simulink model "generalModelForErrorsNEW"  (R2016b)
settings: Solver=ode15s  StartTime=0  StopTime=3500  FixedStep=0.0001  MaxStep=0.001  RelTol=1e-3
values from neighbouring files (symbols this model uses):
  bigpump_const = 1    [run_model.m]
  gain_coef = 4000*10    (= 40000)    [params.m]    (also in run_model.m)
  min_vol = 20    [params.m]
  minipump_const = 0    [run_model.m]
  pipe_diameter = 2    [params.m]
  pressurization = 100000    [params.m]
  pump_speed = 20000    [params.m]
  valve_gain = 0.01    [params.m]
  ws_fault_time = fault_time    [run_model.m]
  ws_sample_time_end_valve_bigpump_in = 0    [run_model.m]
  ws_sample_time_end_valve_bigpump_out = 0    [run_model.m]
  ws_sample_time_end_valve_car_tank = 0    [run_model.m]
  ws_sample_time_end_valve_cartank1_in = 0    [run_model.m]
  ws_sample_time_end_valve_cartank1_out = 0    [run_model.m]
  ws_sample_time_end_valve_cartank2_in = 0    [run_model.m]
  ws_sample_time_end_valve_cartank2_out = 0    [run_model.m]
  ws_sample_time_end_valve_cartank3_in = 0    [run_model.m]
  ws_sample_time_end_valve_cartank3_out = 0    [run_model.m]
  ws_sample_time_end_valve_general_tank = 0    [run_model.m]
  ws_sample_time_end_valve_minipump_in = 0    [run_model.m]
  ws_sample_time_end_valve_minipump_out = 0    [run_model.m]
undefined symbols (not defined in the file or in its folder): sigbuilder_block
libraries: sh_lib x61, nesl_utility x34, fl_lib x32, powerlib_meascontrol x2
(part 2 of 2)

== system generalModelForErrorsNEW/Bigpump/Valve Control3 ==
  In1 : Inport
  Constant : Constant  Value=ws_sample_time_end_valve_bigpump_out
  Logical Operator : Logic  AllPortsSameDT=off  OutDataTypeStr=boolean
  Product : Product
  S2PS1 : nesl_utility/Simulink-PS Converter  PhysicalDomain=network_engine_domain  SubClassName=ps_input  LeftPortType=input  RightPortType=output  PseudoPeriodic=off  Frequencies=[]  NoiseDistribution=none  NoiseParameters=[]  Unit=1  AffineConversion=off  InputFiltering=off  SimscapeFilterOrder=1  InputFilterTimeConstant=.001  UdotUserProvided=0
  Signal Builder : Subsystem  Tag=STV Subsys  LoadFcn=sigbuilder_block('load');  StartFcn=sigbuilder_block('start');  StopFcn=sigbuilder_block('stop');  ClipboardFcn=sigbuilder_block('clipboard');  mask(Sigbuilder block){tuvar=[0:10]}
      mask help: Simulink:masks:SigbuilderBlock_MD
      mask init:
      | if ~strcmp(get_param(bdroot(gcbh),'SimulationStatus'),'stopped') tuvar = sigbuilder_block('maskInit'); end
      settings: CopyFcn=sigbuilder_block('copy');  DeleteFcn=sigbuilder_block('delete');  ModelCloseFcn=sigbuilder_block('modelClose');  PreSaveFcn=sigbuilder_block('preSave');  PauseFcn=sigbuilder_block('pause');  ContinueFcn=sigbuilder_block('continue');  NameChangeFcn=sigbuilder_block('namechange');  OpenFcn=sigbuilder_block('open',[1024.5 -234 1440 722.25 ]);  CloseFcn=sigbuilder_block('close');
      mask Display: plot(0, 0, 100, 100,[2, 2, 32, 32, 2], [68, 8, 8, 68, 68],[32, 2], [38, 38], [32, 19, 2],[53, 60, 44], [32, 17, 17, 2],[16, 16, 31, 31]);txt = getActiveGroup(gcbh);text(2, 100, txt,'verticalAlignment', 'top');
  Transport Delay : TransportDelay  DelayTime=ws_fault_time
  Valve Actuator : sh_lib/Valves/Valve Actuators/Valve Actuator  valve_stroke=valve_stroke m  time_constant=0.01 s  gain=valve_gain*5 m
  Signal : PMIOPort  Port=1  Side=Left
  wires:
  Product/1 -> S2PS1/1
  In1/1 -> Logical Operator/1
  Signal Builder/1(Signal 2) -> Transport Delay/1
  Transport Delay/1 -> Product/2
  Constant/1 -> Logical Operator/2
  Logical Operator/1 -> Product/1
  connections:
  Valve Actuator/RConn1 -- Signal/RConn1
  Valve Actuator/LConn1 -- S2PS1/RConn1

== system generalModelForErrorsNEW/Bigpump/pressure sensor ==
  Hydraulic Pressure Sensor1 : fl_lib/Hydraulic/Hydraulic Sensors/Hydraulic Pressure Sensor
  Hydraulic Reference : fl_lib/Hydraulic/Hydraulic Elements/Hydraulic Reference
  PS-Simulink Converter1 : nesl_utility/PS-Simulink Converter  PhysicalDomain=network_engine_domain  SubClassName=ps_output  LeftPortType=input  RightPortType=output  PseudoPeriodic=off  Frequencies=[]  Unit=1  AffineConversion=off
  Connection Port : PMIOPort  Port=1  Side=Left
  Pressure_valve_bigpump_out : Outport
  wires:
  PS-Simulink Converter1/1 -> Pressure_valve_bigpump_out/1
  connections:
  PS-Simulink Converter1/LConn1 -- Hydraulic Pressure Sensor1/RConn2
  Hydraulic Reference/LConn1 -- Hydraulic Pressure Sensor1/RConn1
  Connection Port/RConn1 -- Hydraulic Pressure Sensor1/LConn1

== system generalModelForErrorsNEW/Bigpump/pressure sensor1 ==
  Hydraulic Pressure Sensor1 : fl_lib/Hydraulic/Hydraulic Sensors/Hydraulic Pressure Sensor
  Hydraulic Reference : fl_lib/Hydraulic/Hydraulic Elements/Hydraulic Reference
  PS-Simulink Converter1 : nesl_utility/PS-Simulink Converter  PhysicalDomain=network_engine_domain  SubClassName=ps_output  LeftPortType=input  RightPortType=output  PseudoPeriodic=off  Frequencies=[]  Unit=1  AffineConversion=off
  Connection Port : PMIOPort  Port=1  Side=Left
  Pressure_valve_bigpump_in : Outport
  wires:
  PS-Simulink Converter1/1 -> Pressure_valve_bigpump_in/1
  connections:
  PS-Simulink Converter1/LConn1 -- Hydraulic Pressure Sensor1/RConn2
  Hydraulic Reference/LConn1 -- Hydraulic Pressure Sensor1/RConn1
  Connection Port/RConn1 -- Hydraulic Pressure Sensor1/LConn1

== system generalModelForErrorsNEW/Car_Tank/Valve Control ==
  In1 : Inport
  Constant : Constant  Value=ws_sample_time_end_valve_car_tank
  Logical Operator : Logic  AllPortsSameDT=off  OutDataTypeStr=boolean
  Product : Product
  S2PS1 : nesl_utility/Simulink-PS Converter  PhysicalDomain=network_engine_domain  SubClassName=ps_input  LeftPortType=input  RightPortType=output  PseudoPeriodic=off  Frequencies=[]  NoiseDistribution=none  NoiseParameters=[]  Unit=1  AffineConversion=off  InputFiltering=off  SimscapeFilterOrder=1  InputFilterTimeConstant=.001  UdotUserProvided=0
  Scope : Scope
  Scope1 : Scope
  Signal Builder : Subsystem  Tag=STV Subsys  LoadFcn=sigbuilder_block('load');  StartFcn=sigbuilder_block('start');  StopFcn=sigbuilder_block('stop');  ClipboardFcn=sigbuilder_block('clipboard');  mask(Sigbuilder block){tuvar=[0:10]}
      mask help: Simulink:masks:SigbuilderBlock_MD
      mask init:
      | if ~strcmp(get_param(bdroot(gcbh),'SimulationStatus'),'stopped') tuvar = sigbuilder_block('maskInit'); end
      settings: CopyFcn=sigbuilder_block('copy');  DeleteFcn=sigbuilder_block('delete');  ModelCloseFcn=sigbuilder_block('modelClose');  PreSaveFcn=sigbuilder_block('preSave');  PauseFcn=sigbuilder_block('pause');  ContinueFcn=sigbuilder_block('continue');  NameChangeFcn=sigbuilder_block('namechange');  OpenFcn=sigbuilder_block('open',[1024.5 -234 1440 722.25 ]);  CloseFcn=sigbuilder_block('close');
      mask Display: plot(0, 0, 100, 100,[2, 2, 32, 32, 2], [68, 8, 8, 68, 68],[32, 2], [38, 38], [32, 19, 2],[53, 60, 44], [32, 17, 17, 2],[16, 16, 31, 31]);txt = getActiveGroup(gcbh);text(2, 100, txt,'verticalAlignment', 'top');
  Transport Delay : TransportDelay  DelayTime=ws_fault_time
  Valve Actuator : sh_lib/Valves/Valve Actuators/Valve Actuator  valve_stroke=valve_stroke m  time_constant=0.01 s  gain=valve_gain*5 m
  Signal : PMIOPort  Port=1  Side=Left
  wires:
  Product/1 -> Scope1/1, S2PS1/1
  Signal Builder/1(Signal 2) -> Transport Delay/1
  Transport Delay/1 -> Product/2
  In1/1 -> Logical Operator/1
  Constant/1 -> Logical Operator/2
  Logical Operator/1 -> Scope/1, Product/1
  connections:
  Valve Actuator/RConn1 -- Signal/RConn1
  Valve Actuator/LConn1 -- S2PS1/RConn1

== system generalModelForErrorsNEW/General_TANK/Valve Control2 ==
  In1 : Inport
  Constant : Constant  Value=ws_sample_time_end_valve_general_tank
  Logical Operator : Logic  AllPortsSameDT=off  OutDataTypeStr=boolean
  Product : Product
  S2PS1 : nesl_utility/Simulink-PS Converter  PhysicalDomain=network_engine_domain  SubClassName=ps_input  LeftPortType=input  RightPortType=output  PseudoPeriodic=off  Frequencies=[]  NoiseDistribution=none  NoiseParameters=[]  Unit=1  AffineConversion=off  InputFiltering=off  SimscapeFilterOrder=1  InputFilterTimeConstant=.001  UdotUserProvided=0
  Signal Builder : Subsystem  Tag=STV Subsys  LoadFcn=sigbuilder_block('load');  StartFcn=sigbuilder_block('start');  StopFcn=sigbuilder_block('stop');  ClipboardFcn=sigbuilder_block('clipboard');  mask(Sigbuilder block){tuvar=[0:10]}
      mask help: Simulink:masks:SigbuilderBlock_MD
      mask init:
      | if ~strcmp(get_param(bdroot(gcbh),'SimulationStatus'),'stopped') tuvar = sigbuilder_block('maskInit'); end
      settings: CopyFcn=sigbuilder_block('copy');  DeleteFcn=sigbuilder_block('delete');  ModelCloseFcn=sigbuilder_block('modelClose');  PreSaveFcn=sigbuilder_block('preSave');  PauseFcn=sigbuilder_block('pause');  ContinueFcn=sigbuilder_block('continue');  NameChangeFcn=sigbuilder_block('namechange');  OpenFcn=sigbuilder_block('open',[1024.5 -234 1440 722.25 ]);  CloseFcn=sigbuilder_block('close');
      mask Display: plot(0, 0, 100, 100,[2, 2, 32, 32, 2], [68, 8, 8, 68, 68],[32, 2], [38, 38], [32, 19, 2],[53, 60, 44], [32, 17, 17, 2],[16, 16, 31, 31]);txt = getActiveGroup(gcbh);text(2, 100, txt,'verticalAlignment', 'top');
  Transport Delay : TransportDelay  DelayTime=ws_fault_time
  Valve Actuator : sh_lib/Valves/Valve Actuators/Valve Actuator  valve_stroke=valve_stroke m  time_constant=0.01 s  gain=valve_gain*5 m
  Signal : PMIOPort  Port=1  Side=Left
  wires:
  Product/1 -> S2PS1/1
  In1/1 -> Logical Operator/1
  Signal Builder/1(Signal 2) -> Transport Delay/1
  Transport Delay/1 -> Product/2
  Constant/1 -> Logical Operator/2
  Logical Operator/1 -> Product/1
  connections:
  Valve Actuator/RConn1 -- Signal/RConn1
  Valve Actuator/LConn1 -- S2PS1/RConn1

== system generalModelForErrorsNEW/Tank1/Valve Control1 ==
  In1 : Inport
  Constant : Constant  Value=ws_sample_time_end_valve_cartank1_in
  Logical Operator : Logic  AllPortsSameDT=off  OutDataTypeStr=boolean
  Product : Product
  S2PS1 : nesl_utility/Simulink-PS Converter  PhysicalDomain=network_engine_domain  SubClassName=ps_input  LeftPortType=input  RightPortType=output  PseudoPeriodic=off  Frequencies=[]  NoiseDistribution=none  NoiseParameters=[]  Unit=1  AffineConversion=off  InputFiltering=off  SimscapeFilterOrder=1  InputFilterTimeConstant=.001  UdotUserProvided=0
  Signal Builder : Subsystem  Tag=STV Subsys  LoadFcn=sigbuilder_block('load');  StartFcn=sigbuilder_block('start');  StopFcn=sigbuilder_block('stop');  ClipboardFcn=sigbuilder_block('clipboard');  mask(Sigbuilder block){tuvar=[0:10]}
      mask help: Simulink:masks:SigbuilderBlock_MD
      mask init:
      | if ~strcmp(get_param(bdroot(gcbh),'SimulationStatus'),'stopped') tuvar = sigbuilder_block('maskInit'); end
      settings: CopyFcn=sigbuilder_block('copy');  DeleteFcn=sigbuilder_block('delete');  ModelCloseFcn=sigbuilder_block('modelClose');  PreSaveFcn=sigbuilder_block('preSave');  PauseFcn=sigbuilder_block('pause');  ContinueFcn=sigbuilder_block('continue');  NameChangeFcn=sigbuilder_block('namechange');  OpenFcn=sigbuilder_block('open',[1024.5 -234 1440 722.25 ]);  CloseFcn=sigbuilder_block('close');
      mask Display: plot(0, 0, 100, 100,[2, 2, 32, 32, 2], [68, 8, 8, 68, 68],[32, 2], [38, 38], [32, 19, 2],[53, 60, 44], [32, 17, 17, 2],[16, 16, 31, 31]);txt = getActiveGroup(gcbh);text(2, 100, txt,'verticalAlignment', 'top');
  Transport Delay : TransportDelay  DelayTime=ws_fault_time
  Valve Actuator : sh_lib/Valves/Valve Actuators/Valve Actuator  valve_stroke=valve_stroke m  time_constant=0.01 s  gain=valve_gain*5 m
  Signal : PMIOPort  Port=1  Side=Left
  wires:
  Product/1 -> S2PS1/1
  In1/1 -> Logical Operator/1
  Signal Builder/1(Signal 2) -> Transport Delay/1
  Transport Delay/1 -> Product/2
  Constant/1 -> Logical Operator/2
  Logical Operator/1 -> Product/1
  connections:
  Valve Actuator/RConn1 -- Signal/RConn1
  Valve Actuator/LConn1 -- S2PS1/RConn1

== system generalModelForErrorsNEW/Tank1/Valve Control2 ==
  In1 : Inport
  Constant : Constant  Value=ws_sample_time_end_valve_cartank1_out
  Logical Operator : Logic  AllPortsSameDT=off  OutDataTypeStr=boolean
  Product : Product
  S2PS1 : nesl_utility/Simulink-PS Converter  PhysicalDomain=network_engine_domain  SubClassName=ps_input  LeftPortType=input  RightPortType=output  PseudoPeriodic=off  Frequencies=[]  NoiseDistribution=none  NoiseParameters=[]  Unit=1  AffineConversion=off  InputFiltering=off  SimscapeFilterOrder=1  InputFilterTimeConstant=.001  UdotUserProvided=0
  Signal Builder : Subsystem  Tag=STV Subsys  LoadFcn=sigbuilder_block('load');  StartFcn=sigbuilder_block('start');  StopFcn=sigbuilder_block('stop');  ClipboardFcn=sigbuilder_block('clipboard');  mask(Sigbuilder block){tuvar=[0:10]}
      mask help: Simulink:masks:SigbuilderBlock_MD
      mask init:
      | if ~strcmp(get_param(bdroot(gcbh),'SimulationStatus'),'stopped') tuvar = sigbuilder_block('maskInit'); end
      settings: CopyFcn=sigbuilder_block('copy');  DeleteFcn=sigbuilder_block('delete');  ModelCloseFcn=sigbuilder_block('modelClose');  PreSaveFcn=sigbuilder_block('preSave');  PauseFcn=sigbuilder_block('pause');  ContinueFcn=sigbuilder_block('continue');  NameChangeFcn=sigbuilder_block('namechange');  OpenFcn=sigbuilder_block('open',[1024.5 -234 1440 722.25 ]);  CloseFcn=sigbuilder_block('close');
      mask Display: plot(0, 0, 100, 100,[2, 2, 32, 32, 2], [68, 8, 8, 68, 68],[32, 2], [38, 38], [32, 19, 2],[53, 60, 44], [32, 17, 17, 2],[16, 16, 31, 31]);txt = getActiveGroup(gcbh);text(2, 100, txt,'verticalAlignment', 'top');
  Transport Delay : TransportDelay  DelayTime=ws_fault_time
  Valve Actuator : sh_lib/Valves/Valve Actuators/Valve Actuator  valve_stroke=valve_stroke m  time_constant=0.01 s  gain=valve_gain*5 m
  Signal : PMIOPort  Port=1  Side=Left
  wires:
  Product/1 -> S2PS1/1
  In1/1 -> Logical Operator/1
  Signal Builder/1(Signal 2) -> Transport Delay/1
  Transport Delay/1 -> Product/2
  Constant/1 -> Logical Operator/2
  Logical Operator/1 -> Product/1
  connections:
  Valve Actuator/RConn1 -- Signal/RConn1
  Valve Actuator/LConn1 -- S2PS1/RConn1

== system generalModelForErrorsNEW/Tank2/Valve Control1 ==
  In1 : Inport
  Constant : Constant  Value=ws_sample_time_end_valve_cartank2_in
  Logical Operator : Logic  AllPortsSameDT=off  OutDataTypeStr=boolean
  Product : Product
  S2PS1 : nesl_utility/Simulink-PS Converter  PhysicalDomain=network_engine_domain  SubClassName=ps_input  LeftPortType=input  RightPortType=output  PseudoPeriodic=off  Frequencies=[]  NoiseDistribution=none  NoiseParameters=[]  Unit=1  AffineConversion=off  InputFiltering=off  SimscapeFilterOrder=1  InputFilterTimeConstant=.001  UdotUserProvided=0
  Signal Builder : Subsystem  Tag=STV Subsys  LoadFcn=sigbuilder_block('load');  StartFcn=sigbuilder_block('start');  StopFcn=sigbuilder_block('stop');  ClipboardFcn=sigbuilder_block('clipboard');  mask(Sigbuilder block){tuvar=[0:10]}
      mask help: Simulink:masks:SigbuilderBlock_MD
      mask init:
      | if ~strcmp(get_param(bdroot(gcbh),'SimulationStatus'),'stopped') tuvar = sigbuilder_block('maskInit'); end
      settings: CopyFcn=sigbuilder_block('copy');  DeleteFcn=sigbuilder_block('delete');  ModelCloseFcn=sigbuilder_block('modelClose');  PreSaveFcn=sigbuilder_block('preSave');  PauseFcn=sigbuilder_block('pause');  ContinueFcn=sigbuilder_block('continue');  NameChangeFcn=sigbuilder_block('namechange');  OpenFcn=sigbuilder_block('open',[1024.5 -234 1440 722.25 ]);  CloseFcn=sigbuilder_block('close');
      mask Display: plot(0, 0, 100, 100,[2, 2, 32, 32, 2], [68, 8, 8, 68, 68],[32, 2], [38, 38], [32, 19, 2],[53, 60, 44], [32, 17, 17, 2],[16, 16, 31, 31]);txt = getActiveGroup(gcbh);text(2, 100, txt,'verticalAlignment', 'top');
  Transport Delay : TransportDelay  DelayTime=ws_fault_time
  Valve Actuator : sh_lib/Valves/Valve Actuators/Valve Actuator  valve_stroke=valve_stroke m  time_constant=0.01 s  gain=valve_gain*5 m
  Signal : PMIOPort  Port=1  Side=Left
  wires:
  Product/1 -> S2PS1/1
  In1/1 -> Logical Operator/1
  Signal Builder/1(Signal 2) -> Transport Delay/1
  Transport Delay/1 -> Product/2
  Constant/1 -> Logical Operator/2
  Logical Operator/1 -> Product/1
  connections:
  Valve Actuator/RConn1 -- Signal/RConn1
  Valve Actuator/LConn1 -- S2PS1/RConn1

== system generalModelForErrorsNEW/Tank2/Valve Control2 ==
  In1 : Inport
  Constant : Constant  Value=ws_sample_time_end_valve_cartank2_out
  Logical Operator : Logic  AllPortsSameDT=off  OutDataTypeStr=boolean
  Product : Product
  S2PS1 : nesl_utility/Simulink-PS Converter  PhysicalDomain=network_engine_domain  SubClassName=ps_input  LeftPortType=input  RightPortType=output  PseudoPeriodic=off  Frequencies=[]  NoiseDistribution=none  NoiseParameters=[]  Unit=1  AffineConversion=off  InputFiltering=off  SimscapeFilterOrder=1  InputFilterTimeConstant=.001  UdotUserProvided=0
  Signal Builder : Subsystem  Tag=STV Subsys  LoadFcn=sigbuilder_block('load');  StartFcn=sigbuilder_block('start');  StopFcn=sigbuilder_block('stop');  ClipboardFcn=sigbuilder_block('clipboard');  mask(Sigbuilder block){tuvar=[0:10]}
      mask help: Simulink:masks:SigbuilderBlock_MD
      mask init:
      | if ~strcmp(get_param(bdroot(gcbh),'SimulationStatus'),'stopped') tuvar = sigbuilder_block('maskInit'); end
      settings: CopyFcn=sigbuilder_block('copy');  DeleteFcn=sigbuilder_block('delete');  ModelCloseFcn=sigbuilder_block('modelClose');  PreSaveFcn=sigbuilder_block('preSave');  PauseFcn=sigbuilder_block('pause');  ContinueFcn=sigbuilder_block('continue');  NameChangeFcn=sigbuilder_block('namechange');  OpenFcn=sigbuilder_block('open',[1024.5 -234 1440 722.25 ]);  CloseFcn=sigbuilder_block('close');
      mask Display: plot(0, 0, 100, 100,[2, 2, 32, 32, 2], [68, 8, 8, 68, 68],[32, 2], [38, 38], [32, 19, 2],[53, 60, 44], [32, 17, 17, 2],[16, 16, 31, 31]);txt = getActiveGroup(gcbh);text(2, 100, txt,'verticalAlignment', 'top');
  Transport Delay : TransportDelay  DelayTime=ws_fault_time
  Valve Actuator : sh_lib/Valves/Valve Actuators/Valve Actuator  valve_stroke=valve_stroke m  time_constant=0.01 s  gain=valve_gain*5 m
  Signal : PMIOPort  Port=1  Side=Left
  wires:
  Product/1 -> S2PS1/1
  In1/1 -> Logical Operator/1
  Signal Builder/1(Signal 2) -> Transport Delay/1
  Transport Delay/1 -> Product/2
  Constant/1 -> Logical Operator/2
  Logical Operator/1 -> Product/1
  connections:
  Valve Actuator/RConn1 -- Signal/RConn1
  Valve Actuator/LConn1 -- S2PS1/RConn1

== system generalModelForErrorsNEW/Tank3/Valve Control1 ==
  In1 : Inport
  Constant : Constant  Value=ws_sample_time_end_valve_cartank3_out
  Logical Operator : Logic  AllPortsSameDT=off  OutDataTypeStr=boolean
  Product : Product
  S2PS1 : nesl_utility/Simulink-PS Converter  PhysicalDomain=network_engine_domain  SubClassName=ps_input  LeftPortType=input  RightPortType=output  PseudoPeriodic=off  Frequencies=[]  NoiseDistribution=none  NoiseParameters=[]  Unit=1  AffineConversion=off  InputFiltering=off  SimscapeFilterOrder=1  InputFilterTimeConstant=.001  UdotUserProvided=0
  Signal Builder : Subsystem  Tag=STV Subsys  LoadFcn=sigbuilder_block('load');  StartFcn=sigbuilder_block('start');  StopFcn=sigbuilder_block('stop');  ClipboardFcn=sigbuilder_block('clipboard');  mask(Sigbuilder block){tuvar=[0:10]}
      mask help: Simulink:masks:SigbuilderBlock_MD
      mask init:
      | if ~strcmp(get_param(bdroot(gcbh),'SimulationStatus'),'stopped') tuvar = sigbuilder_block('maskInit'); end
      settings: CopyFcn=sigbuilder_block('copy');  DeleteFcn=sigbuilder_block('delete');  ModelCloseFcn=sigbuilder_block('modelClose');  PreSaveFcn=sigbuilder_block('preSave');  PauseFcn=sigbuilder_block('pause');  ContinueFcn=sigbuilder_block('continue');  NameChangeFcn=sigbuilder_block('namechange');  OpenFcn=sigbuilder_block('open',[1024.5 -234 1440 722.25 ]);  CloseFcn=sigbuilder_block('close');
      mask Display: plot(0, 0, 100, 100,[2, 2, 32, 32, 2], [68, 8, 8, 68, 68],[32, 2], [38, 38], [32, 19, 2],[53, 60, 44], [32, 17, 17, 2],[16, 16, 31, 31]);txt = getActiveGroup(gcbh);text(2, 100, txt,'verticalAlignment', 'top');
  Transport Delay : TransportDelay  DelayTime=ws_fault_time
  Valve Actuator : sh_lib/Valves/Valve Actuators/Valve Actuator  valve_stroke=valve_stroke m  time_constant=0.01 s  gain=valve_gain*5 m
  Signal : PMIOPort  Port=1  Side=Left
  wires:
  Product/1 -> S2PS1/1
  In1/1 -> Logical Operator/1
  Signal Builder/1(Signal 2) -> Transport Delay/1
  Transport Delay/1 -> Product/2
  Constant/1 -> Logical Operator/2
  Logical Operator/1 -> Product/1
  connections:
  Valve Actuator/RConn1 -- Signal/RConn1
  Valve Actuator/LConn1 -- S2PS1/RConn1

== system generalModelForErrorsNEW/Tank3/Valve Control2 ==
  In1 : Inport
  Constant : Constant  Value=ws_sample_time_end_valve_cartank3_in
  Logical Operator : Logic  AllPortsSameDT=off  OutDataTypeStr=boolean
  Product : Product
  S2PS1 : nesl_utility/Simulink-PS Converter  PhysicalDomain=network_engine_domain  SubClassName=ps_input  LeftPortType=input  RightPortType=output  PseudoPeriodic=off  Frequencies=[]  NoiseDistribution=none  NoiseParameters=[]  Unit=1  AffineConversion=off  InputFiltering=off  SimscapeFilterOrder=1  InputFilterTimeConstant=.001  UdotUserProvided=0
  Signal Builder : Subsystem  Tag=STV Subsys  LoadFcn=sigbuilder_block('load');  StartFcn=sigbuilder_block('start');  StopFcn=sigbuilder_block('stop');  ClipboardFcn=sigbuilder_block('clipboard');  mask(Sigbuilder block){tuvar=[0:10]}
      mask help: Simulink:masks:SigbuilderBlock_MD
      mask init:
      | if ~strcmp(get_param(bdroot(gcbh),'SimulationStatus'),'stopped') tuvar = sigbuilder_block('maskInit'); end
      settings: CopyFcn=sigbuilder_block('copy');  DeleteFcn=sigbuilder_block('delete');  ModelCloseFcn=sigbuilder_block('modelClose');  PreSaveFcn=sigbuilder_block('preSave');  PauseFcn=sigbuilder_block('pause');  ContinueFcn=sigbuilder_block('continue');  NameChangeFcn=sigbuilder_block('namechange');  OpenFcn=sigbuilder_block('open',[1024.5 -234 1440 722.25 ]);  CloseFcn=sigbuilder_block('close');
      mask Display: plot(0, 0, 100, 100,[2, 2, 32, 32, 2], [68, 8, 8, 68, 68],[32, 2], [38, 38], [32, 19, 2],[53, 60, 44], [32, 17, 17, 2],[16, 16, 31, 31]);txt = getActiveGroup(gcbh);text(2, 100, txt,'verticalAlignment', 'top');
  Transport Delay : TransportDelay  DelayTime=ws_fault_time
  Valve Actuator : sh_lib/Valves/Valve Actuators/Valve Actuator  valve_stroke=valve_stroke m  time_constant=0.01 s  gain=valve_gain*5 m
  Signal : PMIOPort  Port=1  Side=Left
  wires:
  Product/1 -> S2PS1/1
  In1/1 -> Logical Operator/1
  Signal Builder/1(Signal 2) -> Transport Delay/1
  Transport Delay/1 -> Product/2
  Constant/1 -> Logical Operator/2
  Logical Operator/1 -> Product/1
  connections:
  Valve Actuator/RConn1 -- Signal/RConn1
  Valve Actuator/LConn1 -- S2PS1/RConn1

== system generalModelForErrorsNEW/minipump/Pressure sensor1 ==
  Hydraulic Pressure Sensor1 : fl_lib/Hydraulic/Hydraulic Sensors/Hydraulic Pressure Sensor
  Hydraulic Reference : fl_lib/Hydraulic/Hydraulic Elements/Hydraulic Reference
  PS-Simulink Converter1 : nesl_utility/PS-Simulink Converter  PhysicalDomain=network_engine_domain  SubClassName=ps_output  LeftPortType=input  RightPortType=output  PseudoPeriodic=off  Frequencies=[]  Unit=1  AffineConversion=off
  Connection Port : PMIOPort  Port=1  Side=Left
  Pressure_valve_pump_out : Outport
  wires:
  PS-Simulink Converter1/1 -> Pressure_valve_pump_out/1
  connections:
  PS-Simulink Converter1/LConn1 -- Hydraulic Pressure Sensor1/RConn2
  Hydraulic Reference/LConn1 -- Hydraulic Pressure Sensor1/RConn1
  Connection Port/RConn1 -- Hydraulic Pressure Sensor1/LConn1

== system generalModelForErrorsNEW/minipump/Pressure sensor2 ==
  Hydraulic Pressure Sensor1 : fl_lib/Hydraulic/Hydraulic Sensors/Hydraulic Pressure Sensor
  Hydraulic Reference : fl_lib/Hydraulic/Hydraulic Elements/Hydraulic Reference
  PS-Simulink Converter1 : nesl_utility/PS-Simulink Converter  PhysicalDomain=network_engine_domain  SubClassName=ps_output  LeftPortType=input  RightPortType=output  PseudoPeriodic=off  Frequencies=[]  Unit=1  AffineConversion=off
  Connection Port : PMIOPort  Port=1  Side=Left
  Pressure_valve_pump_in : Outport
  wires:
  PS-Simulink Converter1/1 -> Pressure_valve_pump_in/1
  connections:
  PS-Simulink Converter1/LConn1 -- Hydraulic Pressure Sensor1/RConn2
  Hydraulic Reference/LConn1 -- Hydraulic Pressure Sensor1/RConn1
  Connection Port/RConn1 -- Hydraulic Pressure Sensor1/LConn1

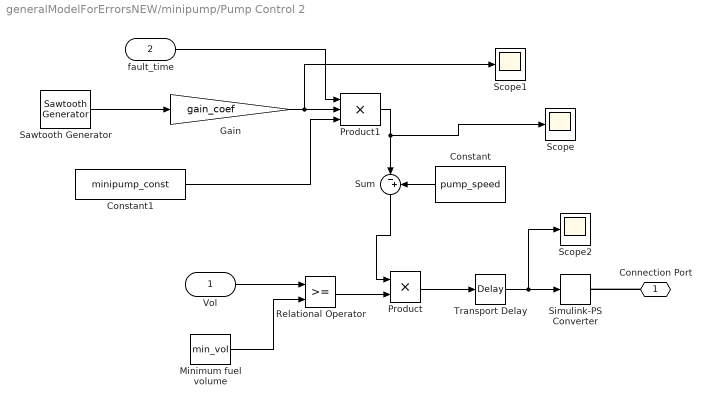
== system generalModelForErrorsNEW/minipump/Pump Control 2 ==
  Vol : Inport
  fault_time : Inport  Port=2
  Constant : Constant  Value=pump_speed
  Constant1 : Constant  Value=minipump_const
  Gain : Gain  Gain=gain_coef
  Minimum fuel volume : Constant  Value=min_vol
  Product : Product  RndMeth=Zero
  Product1 : Product  Inputs=3
  Relational Operator : RelationalOperator  OutDataTypeStr=boolean  RndMeth=Nearest
  Sawtooth Generator : powerlib_meascontrol/Pulse & Signal Generators/Sawtooth Generator  Freq=0.0001  Phase=180  Ts=0
  Scope : Scope
  Scope1 : Scope
  Scope2 : Scope
  Simulink-PS Converter : nesl_utility/Simulink-PS Converter  PhysicalDomain=network_engine_domain  SubClassName=ps_input  LeftPortType=input  RightPortType=output  PseudoPeriodic=off  Frequencies=[]  NoiseDistribution=none  NoiseParameters=[]  Unit=1  AffineConversion=off  InputFiltering=off  SimscapeFilterOrder=1  InputFilterTimeConstant=0.001  UdotUserProvided=1
  Sum : Sum  Inputs=|-+
  Transport Delay : TransportDelay  DelayTime=3
  Connection Port : PMIOPort  Port=1  Side=Left
  wires:
  Sawtooth Generator/1 -> Gain/1
  Transport Delay/1 -> Scope2/1, Simulink-PS Converter/1
  Minimum fuel volume/1 -> Relational Operator/2
  Vol/1 -> Relational Operator/1
  Relational Operator/1 -> Product/2
  Product/1 -> Transport Delay/1
  Constant/1 -> Sum/2
  Sum/1 -> Product/1
  fault_time/1 -> Product1/1
  Gain/1 -> Scope1/1, Product1/2
  Product1/1 -> Scope/1, Sum/1
  Constant1/1 -> Product1/3
  connections:
  Connection Port/RConn1 -- Simulink-PS Converter/RConn1

== system generalModelForErrorsNEW/minipump/Valve Control2 ==
  In1 : Inport
  Constant : Constant  Value=ws_sample_time_end_valve_minipump_in
  Logical Operator : Logic  AllPortsSameDT=off  OutDataTypeStr=boolean
  Product : Product
  S2PS1 : nesl_utility/Simulink-PS Converter  PhysicalDomain=network_engine_domain  SubClassName=ps_input  LeftPortType=input  RightPortType=output  PseudoPeriodic=off  Frequencies=[]  NoiseDistribution=none  NoiseParameters=[]  Unit=1  AffineConversion=off  InputFiltering=off  SimscapeFilterOrder=1  InputFilterTimeConstant=.001  UdotUserProvided=0
  Signal Builder : Subsystem  Tag=STV Subsys  LoadFcn=sigbuilder_block('load');  StartFcn=sigbuilder_block('start');  StopFcn=sigbuilder_block('stop');  ClipboardFcn=sigbuilder_block('clipboard');  mask(Sigbuilder block){tuvar=[0:10]}
      mask help: Simulink:masks:SigbuilderBlock_MD
      mask init:
      | if ~strcmp(get_param(bdroot(gcbh),'SimulationStatus'),'stopped') tuvar = sigbuilder_block('maskInit'); end
      settings: CopyFcn=sigbuilder_block('copy');  DeleteFcn=sigbuilder_block('delete');  ModelCloseFcn=sigbuilder_block('modelClose');  PreSaveFcn=sigbuilder_block('preSave');  PauseFcn=sigbuilder_block('pause');  ContinueFcn=sigbuilder_block('continue');  NameChangeFcn=sigbuilder_block('namechange');  OpenFcn=sigbuilder_block('open',[1024.5 -234 1440 722.25 ]);  CloseFcn=sigbuilder_block('close');
      mask Display: plot(0, 0, 100, 100,[2, 2, 32, 32, 2], [68, 8, 8, 68, 68],[32, 2], [38, 38], [32, 19, 2],[53, 60, 44], [32, 17, 17, 2],[16, 16, 31, 31]);txt = getActiveGroup(gcbh);text(2, 100, txt,'verticalAlignment', 'top');
  Transport Delay : TransportDelay  DelayTime=ws_fault_time
  Valve Actuator : sh_lib/Valves/Valve Actuators/Valve Actuator  valve_stroke=valve_stroke m  time_constant=0.01 s  gain=valve_gain*5 m
  Signal : PMIOPort  Port=1  Side=Left
  wires:
  Product/1 -> S2PS1/1
  In1/1 -> Logical Operator/1
  Signal Builder/1(Signal 2) -> Transport Delay/1
  Transport Delay/1 -> Product/2
  Constant/1 -> Logical Operator/2
  Logical Operator/1 -> Product/1
  connections:
  Valve Actuator/RConn1 -- Signal/RConn1
  Valve Actuator/LConn1 -- S2PS1/RConn1

== system generalModelForErrorsNEW/minipump/Valve Control3 ==
  In1 : Inport
  Constant : Constant  Value=ws_sample_time_end_valve_minipump_out
  Logical Operator : Logic  AllPortsSameDT=off  OutDataTypeStr=boolean
  Product : Product
  S2PS1 : nesl_utility/Simulink-PS Converter  PhysicalDomain=network_engine_domain  SubClassName=ps_input  LeftPortType=input  RightPortType=output  PseudoPeriodic=off  Frequencies=[]  NoiseDistribution=none  NoiseParameters=[]  Unit=1  AffineConversion=off  InputFiltering=off  SimscapeFilterOrder=1  InputFilterTimeConstant=.001  UdotUserProvided=0
  Signal Builder : Subsystem  Tag=STV Subsys  LoadFcn=sigbuilder_block('load');  StartFcn=sigbuilder_block('start');  StopFcn=sigbuilder_block('stop');  ClipboardFcn=sigbuilder_block('clipboard');  mask(Sigbuilder block){tuvar=[0:10]}
      mask help: Simulink:masks:SigbuilderBlock_MD
      mask init:
      | if ~strcmp(get_param(bdroot(gcbh),'SimulationStatus'),'stopped') tuvar = sigbuilder_block('maskInit'); end
      settings: CopyFcn=sigbuilder_block('copy');  DeleteFcn=sigbuilder_block('delete');  ModelCloseFcn=sigbuilder_block('modelClose');  PreSaveFcn=sigbuilder_block('preSave');  PauseFcn=sigbuilder_block('pause');  ContinueFcn=sigbuilder_block('continue');  NameChangeFcn=sigbuilder_block('namechange');  OpenFcn=sigbuilder_block('open',[1024.5 -234 1440 722.25 ]);  CloseFcn=sigbuilder_block('close');
      mask Display: plot(0, 0, 100, 100,[2, 2, 32, 32, 2], [68, 8, 8, 68, 68],[32, 2], [38, 38], [32, 19, 2],[53, 60, 44], [32, 17, 17, 2],[16, 16, 31, 31]);txt = getActiveGroup(gcbh);text(2, 100, txt,'verticalAlignment', 'top');
  Transport Delay : TransportDelay  DelayTime=ws_fault_time
  Valve Actuator : sh_lib/Valves/Valve Actuators/Valve Actuator  valve_stroke=valve_stroke m  time_constant=0.01 s  gain=valve_gain*5 m
  Signal : PMIOPort  Port=1  Side=Left
  wires:
  Product/1 -> S2PS1/1
  In1/1 -> Logical Operator/1
  Signal Builder/1(Signal 2) -> Transport Delay/1
  Transport Delay/1 -> Product/2
  Constant/1 -> Logical Operator/2
  Logical Operator/1 -> Product/1
  connections:
  Valve Actuator/LConn1 -- S2PS1/RConn1
  Valve Actuator/RConn1 -- Signal/RConn1

== system generalModelForErrorsNEW/Bigpump/Valve Control2/Signal Builder ==
  Demux : Demux  Tag=STV Demux  Outputs=1
  FromWs : FromWorkspace  Tag=STV FromWs  VariableName=tuvar  SampleTime=0
      SigBuilderData=|
      | common.afterFinalStr = 'Extrapolate'
      | common.sampleTime = 0
      | dataSet.timeRange = [0 1000]
      | dataSet.name = 'Group 1'
      | sbobj.Groups.Name = 'Group 1'
      | sbobj.Groups.Signals.Name = 'Signal 2'
      | sbobj.Groups.Signals.XData = [0 10 1000]
      | sbobj.Groups.Signals.YData = [-0.949 -0.95 -1.011]
      | sbobj.Groups.TimeRange = [0 1000]
  Signal 2 : Outport  Tag=STV Outport
  wires:
  FromWs/1 -> Demux/1
  Demux/1 -> Signal 2/1

== system generalModelForErrorsNEW/Bigpump/Valve Control3/Signal Builder ==
  Demux : Demux  Tag=STV Demux  Outputs=1
  FromWs : FromWorkspace  Tag=STV FromWs  VariableName=tuvar  SampleTime=0
      SigBuilderData=|
      | common.afterFinalStr = 'Extrapolate'
      | common.sampleTime = 0
      | dataSet.timeRange = [0 1000]
      | dataSet.name = 'Group 1'
      | sbobj.Groups.Name = 'Group 1'
      | sbobj.Groups.Signals.Name = 'Signal 2'
      | sbobj.Groups.Signals.XData = [0 10 1000]
      | sbobj.Groups.Signals.YData = [-0.949 -0.95 -1.011]
      | sbobj.Groups.TimeRange = [0 1000]
  Signal 2 : Outport  Tag=STV Outport
  wires:
  FromWs/1 -> Demux/1
  Demux/1 -> Signal 2/1

== system generalModelForErrorsNEW/Car_Tank/Valve Control/Signal Builder ==
  Demux : Demux  Tag=STV Demux  Outputs=1
  FromWs : FromWorkspace  Tag=STV FromWs  VariableName=tuvar  SampleTime=0
      SigBuilderData=|
      | common.afterFinalStr = 'Extrapolate'
      | common.sampleTime = 0
      | dataSet.timeRange = [0 1000]
      | dataSet.name = 'Group 1'
      | sbobj.Groups.Name = 'Group 1'
      | sbobj.Groups.Signals.Name = 'Signal 2'
      | sbobj.Groups.Signals.XData = [0 10 1000]
      | sbobj.Groups.Signals.YData = [-0.949 -0.95 -1.011]
      | sbobj.Groups.TimeRange = [0 1000]
  Signal 2 : Outport  Tag=STV Outport
  wires:
  FromWs/1 -> Demux/1
  Demux/1 -> Signal 2/1

== system generalModelForErrorsNEW/General_TANK/Valve Control2/Signal Builder ==
  Demux : Demux  Tag=STV Demux  Outputs=1
  FromWs : FromWorkspace  Tag=STV FromWs  VariableName=tuvar  SampleTime=0
      SigBuilderData=|
      | common.afterFinalStr = 'Extrapolate'
      | common.sampleTime = 0
      | dataSet.timeRange = [0 1000]
      | dataSet.name = 'Group 1'
      | sbobj.Groups.Name = 'Group 1'
      | sbobj.Groups.Signals.Name = 'Signal 2'
      | sbobj.Groups.Signals.XData = [0 10 1000]
      | sbobj.Groups.Signals.YData = [-0.949 -0.95 -1.011]
      | sbobj.Groups.TimeRange = [0 1000]
  Signal 2 : Outport  Tag=STV Outport
  wires:
  FromWs/1 -> Demux/1
  Demux/1 -> Signal 2/1

== system generalModelForErrorsNEW/Tank1/Valve Control1/Signal Builder ==
  Demux : Demux  Tag=STV Demux  Outputs=1
  FromWs : FromWorkspace  Tag=STV FromWs  VariableName=tuvar  SampleTime=0
      SigBuilderData=|
      | common.afterFinalStr = 'Extrapolate'
      | common.sampleTime = 0
      | dataSet.timeRange = [0 1000]
      | dataSet.name = 'Group 1'
      | sbobj.Groups.Name = 'Group 1'
      | sbobj.Groups.Signals.Name = 'Signal 2'
      | sbobj.Groups.Signals.XData = [0 10 1000]
      | sbobj.Groups.Signals.YData = [-0.949 -0.95 -1.011]
      | sbobj.Groups.TimeRange = [0 1000]
  Signal 2 : Outport  Tag=STV Outport
  wires:
  FromWs/1 -> Demux/1
  Demux/1 -> Signal 2/1

== system generalModelForErrorsNEW/Tank1/Valve Control2/Signal Builder ==
  Demux : Demux  Tag=STV Demux  Outputs=1
  FromWs : FromWorkspace  Tag=STV FromWs  VariableName=tuvar  SampleTime=0
      SigBuilderData=|
      | common.afterFinalStr = 'Extrapolate'
      | common.sampleTime = 0
      | dataSet.timeRange = [0 1000]
      | dataSet.name = 'Group 1'
      | sbobj.Groups.Name = 'Group 1'
      | sbobj.Groups.Signals.Name = 'Signal 2'
      | sbobj.Groups.Signals.XData = [0 10 1000]
      | sbobj.Groups.Signals.YData = [-0.949 -0.95 -1.011]
      | sbobj.Groups.TimeRange = [0 1000]
  Signal 2 : Outport  Tag=STV Outport
  wires:
  FromWs/1 -> Demux/1
  Demux/1 -> Signal 2/1

== system generalModelForErrorsNEW/Tank2/Valve Control1/Signal Builder ==
  Demux : Demux  Tag=STV Demux  Outputs=1
  FromWs : FromWorkspace  Tag=STV FromWs  VariableName=tuvar  SampleTime=0
      SigBuilderData=|
      | common.afterFinalStr = 'Extrapolate'
      | common.sampleTime = 0
      | dataSet.timeRange = [0 1000]
      | dataSet.name = 'Group 1'
      | sbobj.Groups.Name = 'Group 1'
      | sbobj.Groups.Signals.Name = 'Signal 2'
      | sbobj.Groups.Signals.XData = [0 10 1000]
      | sbobj.Groups.Signals.YData = [-0.949 -0.95 -1.011]
      | sbobj.Groups.TimeRange = [0 1000]
  Signal 2 : Outport  Tag=STV Outport
  wires:
  FromWs/1 -> Demux/1
  Demux/1 -> Signal 2/1

== system generalModelForErrorsNEW/Tank2/Valve Control2/Signal Builder ==
  Demux : Demux  Tag=STV Demux  Outputs=1
  FromWs : FromWorkspace  Tag=STV FromWs  VariableName=tuvar  SampleTime=0
      SigBuilderData=|
      | common.afterFinalStr = 'Extrapolate'
      | common.sampleTime = 0
      | dataSet.timeRange = [0 1000]
      | dataSet.name = 'Group 1'
      | sbobj.Groups.Name = 'Group 1'
      | sbobj.Groups.Signals.Name = 'Signal 2'
      | sbobj.Groups.Signals.XData = [0 10 1000]
      | sbobj.Groups.Signals.YData = [-0.949 -0.95 -1.011]
      | sbobj.Groups.TimeRange = [0 1000]
  Signal 2 : Outport  Tag=STV Outport
  wires:
  FromWs/1 -> Demux/1
  Demux/1 -> Signal 2/1

== system generalModelForErrorsNEW/Tank3/Valve Control1/Signal Builder ==
  Demux : Demux  Tag=STV Demux  Outputs=1
  FromWs : FromWorkspace  Tag=STV FromWs  VariableName=tuvar  SampleTime=0
      SigBuilderData=|
      | common.afterFinalStr = 'Extrapolate'
      | common.sampleTime = 0
      | dataSet.timeRange = [0 1000]
      | dataSet.name = 'Group 1'
      | sbobj.Groups.Name = 'Group 1'
      | sbobj.Groups.Signals.Name = 'Signal 2'
      | sbobj.Groups.Signals.XData = [0 10 1000]
      | sbobj.Groups.Signals.YData = [-0.949 -0.95 -1.011]
      | sbobj.Groups.TimeRange = [0 1000]
  Signal 2 : Outport  Tag=STV Outport
  wires:
  FromWs/1 -> Demux/1
  Demux/1 -> Signal 2/1

== system generalModelForErrorsNEW/Tank3/Valve Control2/Signal Builder ==
  Demux : Demux  Tag=STV Demux  Outputs=1
  FromWs : FromWorkspace  Tag=STV FromWs  VariableName=tuvar  SampleTime=0
      SigBuilderData=|
      | common.afterFinalStr = 'Extrapolate'
      | common.sampleTime = 0
      | dataSet.timeRange = [0 1000]
      | dataSet.name = 'Group 1'
      | sbobj.Groups.Name = 'Group 1'
      | sbobj.Groups.Signals.Name = 'Signal 2'
      | sbobj.Groups.Signals.XData = [0 10 1000]
      | sbobj.Groups.Signals.YData = [-0.949 -0.95 -1.011]
      | sbobj.Groups.TimeRange = [0 1000]
  Signal 2 : Outport  Tag=STV Outport
  wires:
  FromWs/1 -> Demux/1
  Demux/1 -> Signal 2/1

== system generalModelForErrorsNEW/minipump/Valve Control2/Signal Builder ==
  Demux : Demux  Tag=STV Demux  Outputs=1
  FromWs : FromWorkspace  Tag=STV FromWs  VariableName=tuvar  SampleTime=0
      SigBuilderData=|
      | common.afterFinalStr = 'Extrapolate'
      | common.sampleTime = 0
      | dataSet.timeRange = [0 1000]
      | dataSet.name = 'Group 1'
      | sbobj.Groups.Name = 'Group 1'
      | sbobj.Groups.Signals.Name = 'Signal 2'
      | sbobj.Groups.Signals.XData = [0 10 1000]
      | sbobj.Groups.Signals.YData = [-0.949 -0.95 -1.011]
      | sbobj.Groups.TimeRange = [0 1000]
  Signal 2 : Outport  Tag=STV Outport
  wires:
  FromWs/1 -> Demux/1
  Demux/1 -> Signal 2/1

== system generalModelForErrorsNEW/minipump/Valve Control3/Signal Builder ==
  Demux : Demux  Tag=STV Demux  Outputs=1
  FromWs : FromWorkspace  Tag=STV FromWs  VariableName=tuvar  SampleTime=0
      SigBuilderData=|
      | common.afterFinalStr = 'Extrapolate'
      | common.sampleTime = 0
      | dataSet.timeRange = [0 1000]
      | dataSet.name = 'Group 1'
      | sbobj.Groups.Name = 'Group 1'
      | sbobj.Groups.Signals.Name = 'Signal 2'
      | sbobj.Groups.Signals.XData = [0 10 1000]
      | sbobj.Groups.Signals.YData = [-0.949 -0.95 -1.011]
      | sbobj.Groups.TimeRange = [0 1000]
  Signal 2 : Outport  Tag=STV Outport
  wires:
  FromWs/1 -> Demux/1
  Demux/1 -> Signal 2/1
